simulink model "twolevel_parallel"  (R2016a)
settings: Solver=VariableStepAuto  StartTime=0.0  StopTime=stop_time  RelTol=1e-3
values from neighbouring files (symbols this model uses):
  DCLINK_Cap = 0.6*capacitorsabiti/sw_frequency    (= 0.0016)    [loadvariation.m]    (also in twolevel_parallel_analysis.m = 0.0001)
  Ef = Vln_rms*cos(Load_Angle)    [loadvariation.m]    (also in twolevel_parallel_analysis.m)
  intangle1 = 0    [loadvariation.m]    (also in twolevel_parallel_analysis.m)
  intangle2 = intangle1 + interleaving_angle    (= 360)    [loadvariation.m]    (also in twolevel_parallel_analysis.m = 180)
  Load_Angle = acos(Load_Power_Factor)    [loadvariation.m]    (also in twolevel_parallel_analysis.m)
  Ls = Xs/ref_frequency    [loadvariation.m]    (also in twolevel_parallel_analysis.m = n*Xs/ref_frequency)
  ma = 0.9    [loadvariation.m]    (also in twolevel_parallel_analysis.m)
  ref_frequency = 2*pi*50    (= 314.159265359)    [loadvariation.m]    (also in twolevel_parallel_analysis.m)
  Sampling_time = 1/(20*50000)    (= 1e-06)    [loadvariation.m]    (also in twolevel_parallel_analysis.m = 2.43902439024e-05)
  Vin = DC_Voltage_Source + Rin*(Load_Real_Power/DC_Voltage_Source)    (= 554.814814815)    [loadvariation.m]    (also in twolevel_parallel_analysis.m)
undefined symbols (not defined in the file or in its folder): Rload
libraries: powerlib x37, powerlib_meascontrol x23, simulink x12
settings Model: Creator=hakan  LastModifiedBy=hakan

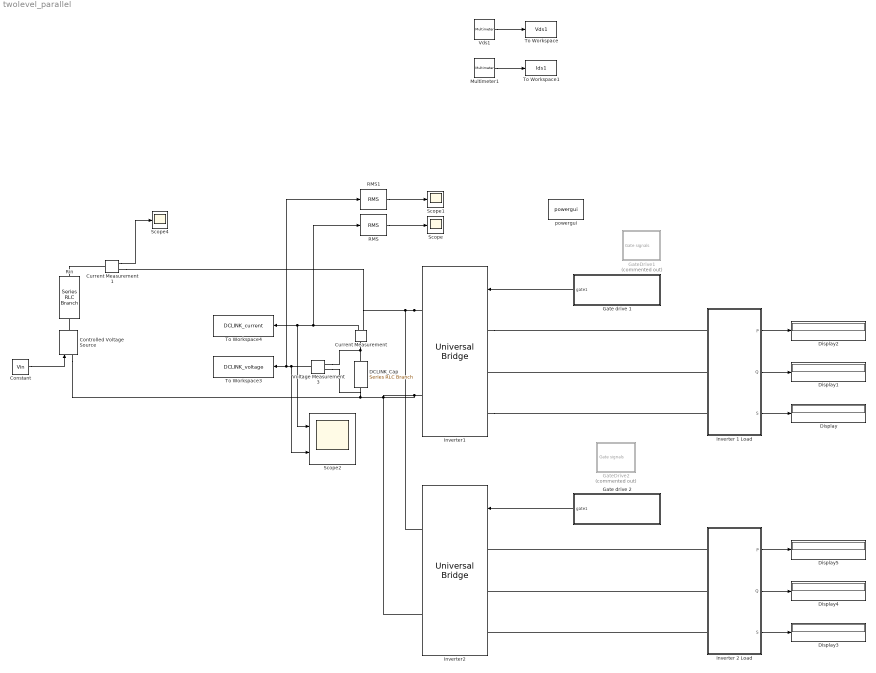
== system twolevel_parallel ==
  Constant : Constant  Value=Vin
  Controlled Voltage Source : powerlib/Electrical Sources/Controlled Voltage Source  Initialize=on  Source_Type=DC  Amplitude=0  Phase=0  Frequency=0  Measurements=None
  Current Measurement : powerlib/Measurements/Current Measurement  PhasorSimulation=off  OutputType=Complex  PSBequivalent=0
  Current Measurement1 : powerlib/Measurements/Current Measurement  PhasorSimulation=off  OutputType=Complex  PSBequivalent=0
  DCLINK_Cap : powerlib/Elements/Series RLC Branch  LConnTagsString=__new0  RConnTagsString=__new0  BranchType=C  Resistance=1  Inductance=1e-3  SetiL0=off  InitialCurrent=0  Capacitance=DCLINK_Cap  Setx0=on  InitialVoltage=540  Measurements=None
  Display{,1..5} (6 alike) : Display
  Gate drive 1 : Subsystem
  Gate drive 2 : Subsystem
  GateDrive1 : Subsystem  Commented=on
  GateDrive2 : Subsystem  Commented=on
  Inverter 1 Load : Subsystem
  Inverter 2 Load : Subsystem
  Inverter1 : powerlib/Power Electronics/Universal Bridge  Arms=3  SnubberResistance=1e5  SnubberCapacitance=inf  Device=IGBT / Diodes  Ron=0.65e-3  Lon=0  ForwardVoltages="[  0  0  ]"  ForwardVoltage=0  GTOparameters=[ 10e-6 , 20e-6 ]  IGBTparameters=[ 1e-6 , 2e-6 ]  Measurements=All voltages and currents  Measurements_2=None  converterType=Rectifier
  Inverter2 : powerlib/Power Electronics/Universal Bridge  Arms=3  SnubberResistance=1e5  SnubberCapacitance=inf  Device=IGBT / Diodes  Ron=0.65e-3  Lon=0  ForwardVoltages="[  0  0  ]"  ForwardVoltage=0  GTOparameters=[ 10e-6 , 20e-6 ]  IGBTparameters=[ 1e-6 , 2e-6 ]  Measurements=All voltages and currents  Measurements_2=None  converterType=Rectifier
  Multimeter1 : powerlib/Measurements/Multimeter  PhasorSimulation=off  OutputType=Complex  sel=27  L=32  Gain=1  yselected={'Isw1: Inverter1'};  PSBOutputType=1  PSBequivalent=0  AxesSetting=[0,0.1,-100,100]  Display=0  SavedBlockNames=-11
  RMS : powerlib_meascontrol/Measurements/RMS  TrueRMS=on  Freq=Load_Nominal_Freq  RMSInit=10  Ts=0
  RMS1 : powerlib_meascontrol/Measurements/RMS  TrueRMS=on  Freq=Load_Nominal_Freq  RMSInit=10  Ts=0
  Rin : powerlib/Elements/Series RLC Branch  LConnTagsString=__new0  RConnTagsString=__new0  BranchType=R  Resistance=1  Inductance=1e-3  SetiL0=off  InitialCurrent=0  Capacitance=1000e-6  Setx0=off  InitialVoltage=0  Measurements=None
  Scope : Scope
  Scope1 : Scope
  Scope2 : Scope  NumInputPorts=2
  Scope4 : Scope
  To Workspace : ToWorkspace  VariableName=Vds1  SaveFormat=Timeseries  SampleTime=-1
  To Workspace1 : ToWorkspace  VariableName=Ids1  SaveFormat=Timeseries  SampleTime=-1
  To Workspace3 : ToWorkspace  VariableName=DCLINK_voltage  SaveFormat=Timeseries  SampleTime=-1
  To Workspace4 : ToWorkspace  VariableName=DCLINK_current  SaveFormat=Timeseries  SampleTime=-1
  Vds1 : powerlib/Measurements/Multimeter  PhasorSimulation=off  OutputType=Complex  sel=11  L=32  Gain=1  yselected={'Usw1: Inverter1'};  PSBOutputType=1  PSBequivalent=0  AxesSetting=[0,0.1,-100,100]  Display=0  SavedBlockNames=-11
  Voltage Measurement3 : powerlib/Measurements/Voltage Measurement  PhasorSimulation=off  OutputType=Complex  PSBequivalent=0
  powergui : powerlib/powergui  Priority=1  SimulationMode=Discrete  SolverType=Tustin  SampleTime=Sampling_time  frequency=60  SPID=off  DisableSnubberDevices=off  DisableRonSwitches=off  DisableVfSwitches=off  SwTol=0  DisplayEquations=off  Interpol=off  ExternalGateDelay=off  methode=off  Ts=10  FunctionMessages=off  echomessages=off  HookPort=off  EnableUseOfTLC=off  x0status=blocks  frequencyindice=0  Pbase=100e6  ErrMax=1e-4  Iterations=50  UnitsV=kV  UnitsW=MW  buscounter=0  RestoreLinks=warning  ResistiveCurrentMeasurement=off  Frange=[0:2:500]  Ylog=off  Xlog=on  ShowGrid=off  save=off  variable=ZData  structure=Phase_currents  ZoomFFT=off  StartTime=0.1  cycles=5  DisplayStyle=1  fundamental=50  FreqAxis=off  MaxFrequency=2000  frequencyindicesteady=1  RmsSteady=1  display=off
  wires:
  Constant/1 -> Controlled Voltage Source/1
  Current Measurement/1 -> Scope2/1, To Workspace4/1, RMS/1
  Voltage Measurement3/1 -> Scope2/2, RMS1/1, To Workspace3/1
  Gate drive 2/1(gate1) -> Inverter2/1
  RMS/1 -> Scope/1
  RMS1/1 -> Scope1/1
  Current Measurement1/1 -> Scope4/1
  Gate drive 1/1(gate1) -> Inverter1/1
  Inverter 1 Load/1(P) -> Display2/1
  Inverter 1 Load/2(Q) -> Display1/1
  Inverter 1 Load/3(S) -> Display/1
  Inverter 2 Load/1(P) -> Display5/1
  Inverter 2 Load/2(Q) -> Display4/1
  Inverter 2 Load/3(S) -> Display3/1
  Multimeter1/1 -> To Workspace1/1
  Vds1/1 -> To Workspace/1
  connections:
  Controlled Voltage Source/RConn1 -- Rin/RConn1
  Inverter1/RConn1 -- Inverter2/RConn1 -- Current Measurement1/RConn1 -- Current Measurement/RConn1
  Inverter1/RConn2 -- Inverter2/RConn2 -- Controlled Voltage Source/LConn1 -- DCLINK_Cap/RConn1 -- Voltage Measurement3/LConn2
  Current Measurement/LConn1 -- DCLINK_Cap/LConn1 -- Voltage Measurement3/LConn1
  Inverter1/LConn1 -- Inverter 1 Load/LConn1
  Inverter 1 Load/LConn2 -- Inverter1/LConn2
  Inverter1/LConn3 -- Inverter 1 Load/LConn3
  Inverter 2 Load/LConn1 -- Inverter2/LConn1
  Inverter 2 Load/LConn3 -- Inverter2/LConn3
  Inverter 2 Load/LConn2 -- Inverter2/LConn2
  Rin/LConn1 -- Current Measurement1/LConn1

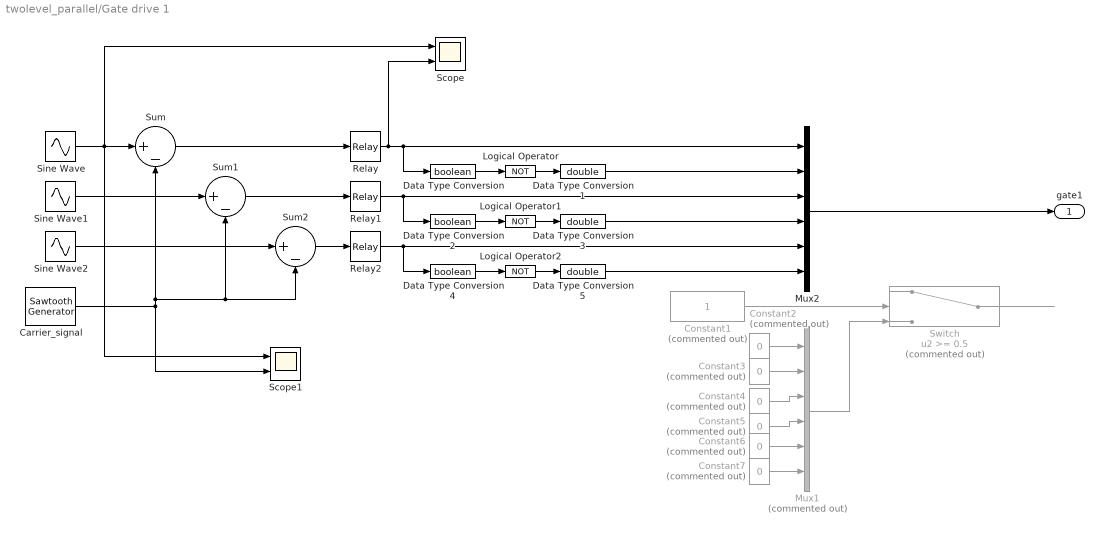
== system twolevel_parallel/Gate drive 1 ==
  Carrier_signal : powerlib_meascontrol/Pulse & Signal Generators/Sawtooth Generator  Freq=sw_frequency  Phase=intangle1  Ts=0
  Constant1 : Constant  Commented=on
  Constant{2..7} (6 alike) : Constant  Commented=on  Value=0
  Data Type Conversion : DataTypeConversion  OutDataTypeStr=boolean
  Data Type Conversion1 : DataTypeConversion  OutDataTypeStr=double
  Data Type Conversion2 : DataTypeConversion  OutDataTypeStr=boolean
  Data Type Conversion3 : DataTypeConversion  OutDataTypeStr=double
  Data Type Conversion4 : DataTypeConversion  OutDataTypeStr=boolean
  Data Type Conversion5 : DataTypeConversion  OutDataTypeStr=double
  Logical Operator : Logic  Operator=NOT  AllPortsSameDT=off  OutDataTypeStr=boolean
  Logical Operator1 : Logic  Operator=NOT  AllPortsSameDT=off  OutDataTypeStr=boolean
  Logical Operator2 : Logic  Operator=NOT  AllPortsSameDT=off  OutDataTypeStr=boolean
  Mux1 : Mux  Commented=on  Inputs=6
  Mux2 : Mux  Inputs=6
  Relay : Relay
  Relay1 : Relay
  Relay2 : Relay
  Scope : Scope  NumInputPorts=2
  Scope1 : Scope  NumInputPorts=2
  Sine Wave : Sin  Amplitude=ma  Frequency=ref_frequency  Phase=Load_Angle  SampleTime=0
  Sine Wave1 : Sin  Amplitude=ma  Frequency=ref_frequency  Phase=-2*pi/3+Load_Angle  SampleTime=0
  Sine Wave2 : Sin  Amplitude=ma  Frequency=ref_frequency  Phase=2*pi/3+Load_Angle  SampleTime=0
  Sum : Sum  Inputs=|+-
  Sum1 : Sum  Inputs=|+-
  Sum2 : Sum  Inputs=|+-
  Switch : Switch  Commented=on  Threshold=0.5
  gate1 : Outport
  wires:
  Sine Wave/1 -> Scope1/1, Scope/1, Sum/1
  Carrier_signal/1 -> Sum1/2, Sum2/2, Sum/2, Scope1/2
  Sine Wave1/1 -> Sum1/1
  Sine Wave2/1 -> Sum2/1
  Sum/1 -> Relay/1
  Sum1/1 -> Relay1/1
  Sum2/1 -> Relay2/1
  Data Type Conversion/1 -> Logical Operator/1
  Relay/1 -> Scope/2, Data Type Conversion/1, Mux2/1
  Logical Operator/1 -> Data Type Conversion1/1
  Data Type Conversion1/1 -> Mux2/2
  Data Type Conversion2/1 -> Logical Operator1/1
  Relay1/1 -> Data Type Conversion2/1, Mux2/3
  Logical Operator1/1 -> Data Type Conversion3/1
  Data Type Conversion3/1 -> Mux2/4
  Data Type Conversion4/1 -> Logical Operator2/1
  Relay2/1 -> Data Type Conversion4/1, Mux2/5
  Logical Operator2/1 -> Data Type Conversion5/1
  Data Type Conversion5/1 -> Mux2/6
  Constant1/1 -> Switch/2
  Constant2/1 -> Mux1/1
  Constant3/1 -> Mux1/2
  Constant4/1 -> Mux1/3
  Constant5/1 -> Mux1/4
  Constant7/1 -> Mux1/6
  Constant6/1 -> Mux1/5
  Mux1/1 -> Switch/3
  Switch/1 -> ?
  Mux2/1 -> gate1/1

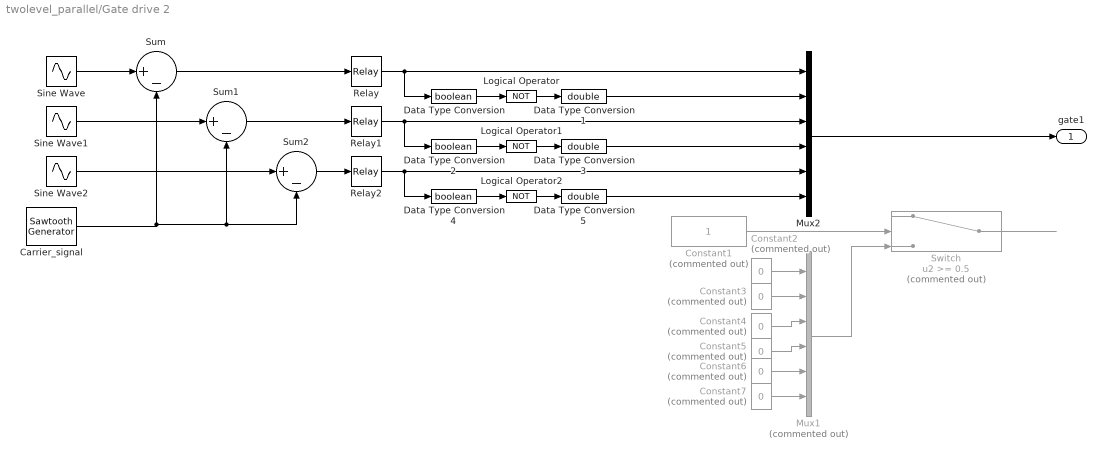
== system twolevel_parallel/Gate drive 2 ==
  Carrier_signal : powerlib_meascontrol/Pulse & Signal Generators/Sawtooth Generator  Freq=sw_frequency  Phase=intangle2  Ts=0
  Constant1 : Constant  Commented=on
  Constant{2..7} (6 alike) : Constant  Commented=on  Value=0
  Data Type Conversion : DataTypeConversion  OutDataTypeStr=boolean
  Data Type Conversion1 : DataTypeConversion  OutDataTypeStr=double
  Data Type Conversion2 : DataTypeConversion  OutDataTypeStr=boolean
  Data Type Conversion3 : DataTypeConversion  OutDataTypeStr=double
  Data Type Conversion4 : DataTypeConversion  OutDataTypeStr=boolean
  Data Type Conversion5 : DataTypeConversion  OutDataTypeStr=double
  Logical Operator : Logic  Operator=NOT  AllPortsSameDT=off  OutDataTypeStr=boolean
  Logical Operator1 : Logic  Operator=NOT  AllPortsSameDT=off  OutDataTypeStr=boolean
  Logical Operator2 : Logic  Operator=NOT  AllPortsSameDT=off  OutDataTypeStr=boolean
  Mux1 : Mux  Commented=on  Inputs=6
  Mux2 : Mux  Inputs=6
  Relay : Relay
  Relay1 : Relay
  Relay2 : Relay
  Sine Wave : Sin  Amplitude=ma  Frequency=ref_frequency  Phase=Load_Angle  SampleTime=0
  Sine Wave1 : Sin  Amplitude=ma  Frequency=ref_frequency  Phase=-2*pi/3+Load_Angle  SampleTime=0
  Sine Wave2 : Sin  Amplitude=ma  Frequency=ref_frequency  Phase=2*pi/3+Load_Angle  SampleTime=0
  Sum : Sum  Inputs=|+-
  Sum1 : Sum  Inputs=|+-
  Sum2 : Sum  Inputs=|+-
  Switch : Switch  Commented=on  Threshold=0.5
  gate1 : Outport
  wires:
  Mux2/1 -> gate1/1
  Switch/1 -> ?
  Mux1/1 -> Switch/3
  Constant6/1 -> Mux1/5
  Constant7/1 -> Mux1/6
  Constant5/1 -> Mux1/4
  Constant4/1 -> Mux1/3
  Constant3/1 -> Mux1/2
  Constant2/1 -> Mux1/1
  Constant1/1 -> Switch/2
  Data Type Conversion5/1 -> Mux2/6
  Logical Operator2/1 -> Data Type Conversion5/1
  Relay2/1 -> Mux2/5, Data Type Conversion4/1
  Data Type Conversion4/1 -> Logical Operator2/1
  Data Type Conversion3/1 -> Mux2/4
  Logical Operator1/1 -> Data Type Conversion3/1
  Relay1/1 -> Mux2/3, Data Type Conversion2/1
  Data Type Conversion2/1 -> Logical Operator1/1
  Data Type Conversion1/1 -> Mux2/2
  Logical Operator/1 -> Data Type Conversion1/1
  Relay/1 -> Mux2/1, Data Type Conversion/1
  Data Type Conversion/1 -> Logical Operator/1
  Sum2/1 -> Relay2/1
  Sum1/1 -> Relay1/1
  Sum/1 -> Relay/1
  Sine Wave2/1 -> Sum2/1
  Sine Wave1/1 -> Sum1/1
  Carrier_signal/1 -> Sum/2, Sum2/2, Sum1/2
  Sine Wave/1 -> Sum/1

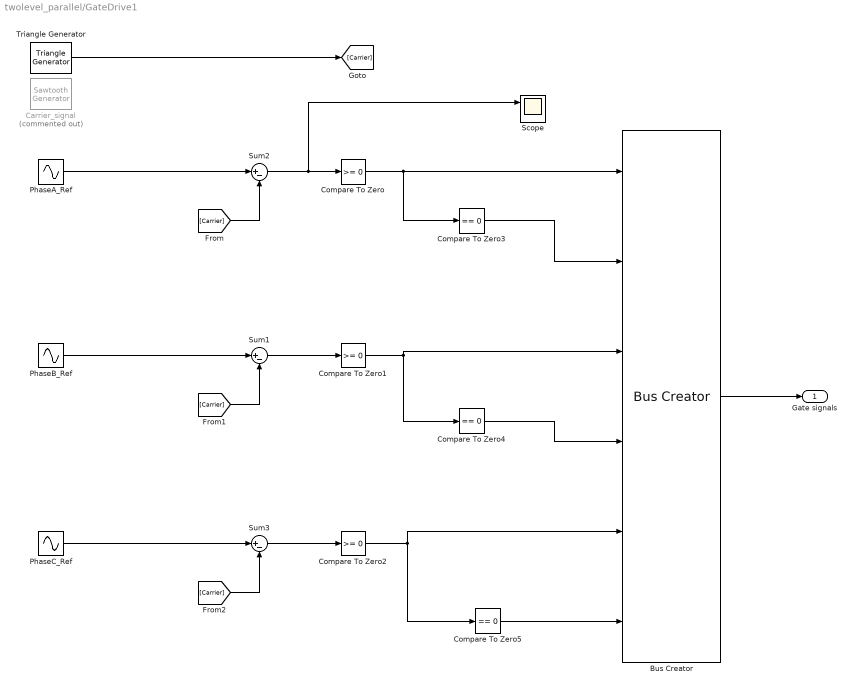
== system twolevel_parallel/GateDrive1 ==
  Bus Creator : BusCreator  Inputs=6
  Carrier_signal : powerlib_meascontrol/Pulse & Signal Generators/Sawtooth Generator  Commented=on  Freq=sw_frequency  Phase=intangle1  Ts=0
  Compare To Zero : simulink/Logic and Bit Operations/Compare To Zero  relop=>=  OutDataTypeStr=boolean  ZeroCross=off
  Compare To Zero1 : simulink/Logic and Bit Operations/Compare To Zero  relop=>=  OutDataTypeStr=boolean  ZeroCross=off
  Compare To Zero2 : simulink/Logic and Bit Operations/Compare To Zero  relop=>=  OutDataTypeStr=boolean  ZeroCross=off
  Compare To Zero3 : simulink/Logic and Bit Operations/Compare To Zero  relop===  OutDataTypeStr=boolean  ZeroCross=off
  Compare To Zero4 : simulink/Logic and Bit Operations/Compare To Zero  relop===  OutDataTypeStr=boolean  ZeroCross=off
  Compare To Zero5 : simulink/Logic and Bit Operations/Compare To Zero  relop===  OutDataTypeStr=boolean  ZeroCross=off
  PhaseA_Ref : Sin  Amplitude=ma  Frequency=ref_frequency  Phase=Load_Angle  SampleTime=0
  PhaseB_Ref : Sin  Amplitude=ma  Frequency=ref_frequency  Phase=-2*pi/3 + Load_Angle  SampleTime=0
  PhaseC_Ref : Sin  Amplitude=ma  Frequency=ref_frequency  Phase=2*pi/3+Load_Angle  SampleTime=0
  Scope : Scope  NumInputPorts=2
  Sum1 : Sum  Inputs=|+-
  Sum2 : Sum  Inputs=|+-
  Sum3 : Sum  Inputs=|+-
  Triangle Generator : powerlib_meascontrol/Pulse & Signal Generators/Triangle Generator  Freq=sw_frequency  Phase=intangle1  Ts=0
  Gate signals : Outport
  wires:
  Triangle Generator/1 -> [Carrier]
  Compare To Zero5/1 -> Bus Creator/6
  Compare To Zero4/1 -> Bus Creator/4
  Compare To Zero3/1 -> Bus Creator/2
  Sum3/1 -> Compare To Zero2/1
  Sum1/1 -> Compare To Zero1/1
  [Carrier] -> Sum3/2
  PhaseC_Ref/1 -> Sum3/1
  Compare To Zero2/1 -> Bus Creator/5, Compare To Zero5/1
  [Carrier] -> Sum1/2
  PhaseB_Ref/1 -> Sum1/1
  Compare To Zero1/1 -> Bus Creator/3, Compare To Zero4/1
  [Carrier] -> Sum2/2
  Sum2/1 -> Scope/1, Compare To Zero/1
  Compare To Zero/1 -> Bus Creator/1, Compare To Zero3/1
  PhaseA_Ref/1 -> Sum2/1
  Bus Creator/1 -> Gate signals/1

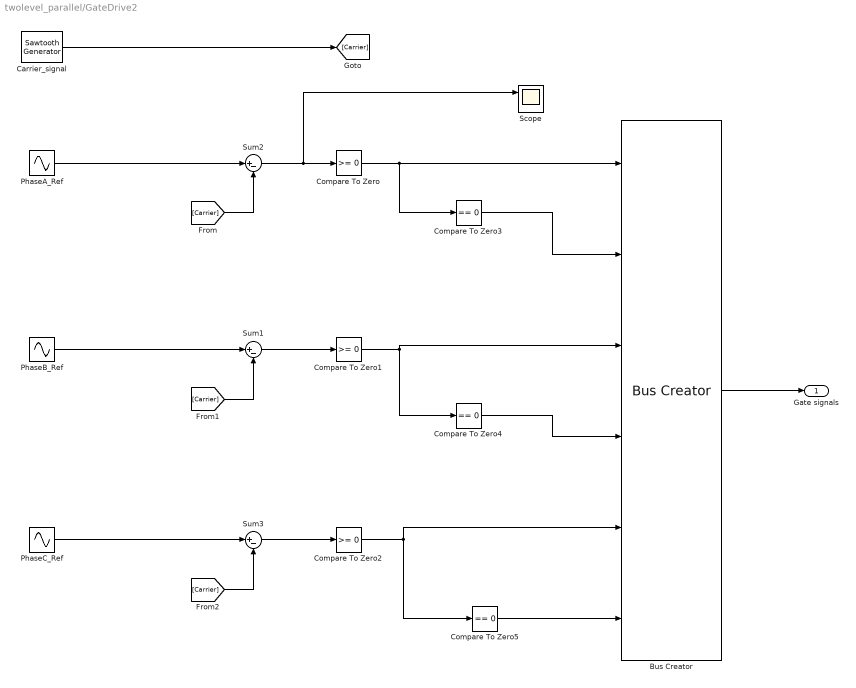
== system twolevel_parallel/GateDrive2 ==
  Bus Creator : BusCreator  Inputs=6
  Carrier_signal : powerlib_meascontrol/Pulse & Signal Generators/Sawtooth Generator  Freq=sw_frequency  Phase=intangle1  Ts=0
  Compare To Zero : simulink/Logic and Bit Operations/Compare To Zero  relop=>=  OutDataTypeStr=boolean  ZeroCross=off
  Compare To Zero1 : simulink/Logic and Bit Operations/Compare To Zero  relop=>=  OutDataTypeStr=boolean  ZeroCross=off
  Compare To Zero2 : simulink/Logic and Bit Operations/Compare To Zero  relop=>=  OutDataTypeStr=boolean  ZeroCross=off
  Compare To Zero3 : simulink/Logic and Bit Operations/Compare To Zero  relop===  OutDataTypeStr=boolean  ZeroCross=off
  Compare To Zero4 : simulink/Logic and Bit Operations/Compare To Zero  relop===  OutDataTypeStr=boolean  ZeroCross=off
  Compare To Zero5 : simulink/Logic and Bit Operations/Compare To Zero  relop===  OutDataTypeStr=boolean  ZeroCross=off
  PhaseA_Ref : Sin  Amplitude=ma  Frequency=ref_frequency  SampleTime=0
  PhaseB_Ref : Sin  Amplitude=ma  Frequency=ref_frequency  Phase=-2*pi/3  SampleTime=0
  PhaseC_Ref : Sin  Amplitude=ma  Frequency=ref_frequency  Phase=2*pi/3  SampleTime=0
  Scope : Scope  NumInputPorts=2
  Sum1 : Sum  Inputs=|+-
  Sum2 : Sum  Inputs=|+-
  Sum3 : Sum  Inputs=|+-
  Gate signals : Outport
  wires:
  Bus Creator/1 -> Gate signals/1
  PhaseA_Ref/1 -> Sum2/1
  Compare To Zero/1 -> Compare To Zero3/1, Bus Creator/1
  Sum2/1 -> Compare To Zero/1, Scope/1
  [Carrier] -> Sum2/2
  Compare To Zero1/1 -> Compare To Zero4/1, Bus Creator/3
  PhaseB_Ref/1 -> Sum1/1
  [Carrier] -> Sum1/2
  Compare To Zero2/1 -> Compare To Zero5/1, Bus Creator/5
  PhaseC_Ref/1 -> Sum3/1
  [Carrier] -> Sum3/2
  Sum1/1 -> Compare To Zero1/1
  Sum3/1 -> Compare To Zero2/1
  Compare To Zero3/1 -> Bus Creator/2
  Compare To Zero4/1 -> Bus Creator/4
  Compare To Zero5/1 -> Bus Creator/6
  Carrier_signal/1 -> [Carrier]

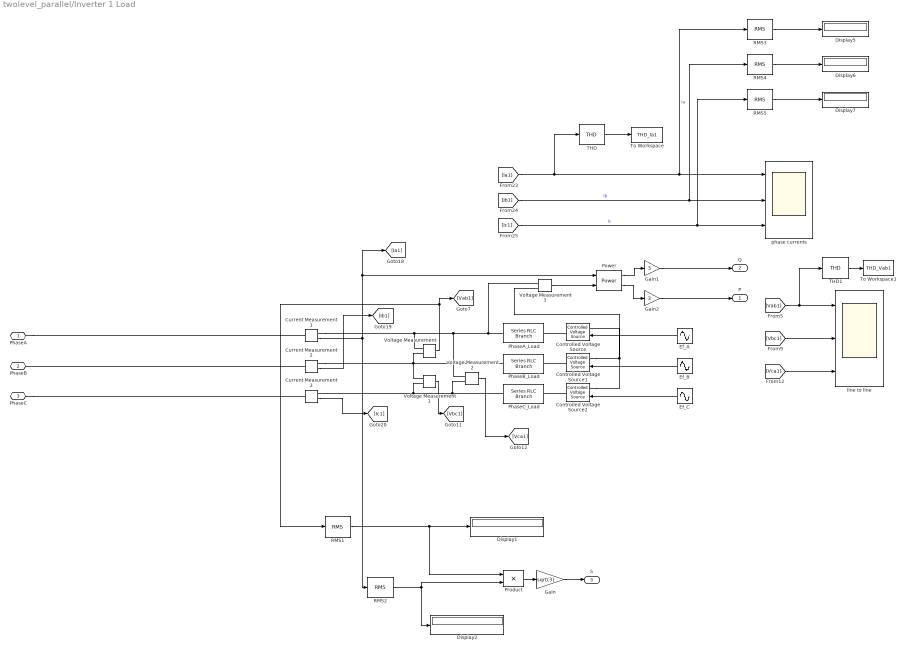
== system twolevel_parallel/Inverter 1 Load ==
  Controlled Voltage Source : powerlib/Electrical Sources/Controlled Voltage Source  Initialize=on  Source_Type=AC  Amplitude=0  Phase=0  Frequency=0  Measurements=None
  Controlled Voltage Source1 : powerlib/Electrical Sources/Controlled Voltage Source  Initialize=on  Source_Type=AC  Amplitude=0  Phase=0  Frequency=0  Measurements=None
  Controlled Voltage Source2 : powerlib/Electrical Sources/Controlled Voltage Source  Initialize=on  Source_Type=AC  Amplitude=0  Phase=0  Frequency=0  Measurements=None
  Current Measurement1 : powerlib/Measurements/Current Measurement  PhasorSimulation=off  OutputType=Complex  PSBequivalent=0
  Current Measurement2 : powerlib/Measurements/Current Measurement  PhasorSimulation=off  OutputType=Complex  PSBequivalent=0
  Current Measurement3 : powerlib/Measurements/Current Measurement  PhasorSimulation=off  OutputType=Complex  PSBequivalent=0
  Display{1..2,5..7} (5 alike) : Display
  Ef_A : Sin  Amplitude=Ef*sqrt(2)  Frequency=ref_frequency  SampleTime=0
  Ef_B : Sin  Amplitude=Ef*sqrt(2)  Frequency=ref_frequency  Phase=-2*pi/3  SampleTime=0
  Ef_C : Sin  Amplitude=Ef*sqrt(2)  Frequency=ref_frequency  Phase=2*pi/3  SampleTime=0
  Gain : Gain  Gain=sqrt(3)
  Gain1 : Gain  Gain=3
  Gain2 : Gain  Gain=3
  PhaseA_Load : powerlib/Elements/Series RLC Branch  LConnTagsString=__new0  RConnTagsString=__new0  BranchType=L  Resistance=Rload  Inductance=Ls  SetiL0=off  InitialCurrent=0  Capacitance=1e-6  Setx0=off  InitialVoltage=0  Measurements=None
  PhaseB_Load : powerlib/Elements/Series RLC Branch  LConnTagsString=__new0  RConnTagsString=__new0  BranchType=L  Resistance=Rload  Inductance=Ls  SetiL0=off  InitialCurrent=0  Capacitance=1e-6  Setx0=off  InitialVoltage=0  Measurements=None
  PhaseC_Load : powerlib/Elements/Series RLC Branch  LConnTagsString=__new0  RConnTagsString=__new0  BranchType=L  Resistance=Rload  Inductance=Ls  SetiL0=off  InitialCurrent=0  Capacitance=1e-6  Setx0=off  InitialVoltage=0  Measurements=None
  Power : powerlib_meascontrol/Measurements/Power  Freq=50  Vinit=[1, 0]  Iinit=[1, 0]  Ts=0
  Product : Product
  RMS1 : powerlib_meascontrol/Measurements/RMS  TrueRMS=off  Freq=Load_Nominal_Freq  RMSInit=120  Ts=0
  RMS{2..5} (4 alike) : powerlib_meascontrol/Measurements/RMS  TrueRMS=on  Freq=Load_Nominal_Freq  RMSInit=120  Ts=0
  THD : powerlib_meascontrol/Measurements/THD  Freq=50  Ts=0
  THD1 : powerlib_meascontrol/Measurements/THD  Freq=50  Ts=0
  To Workspace : ToWorkspace  VariableName=THD_Ia1  SaveFormat=Timeseries  SampleTime=-1
  To Workspace1 : ToWorkspace  VariableName=THD_Vab1  SaveFormat=Timeseries  SampleTime=-1
  Voltage Measurement{,1..3} (4 alike) : powerlib/Measurements/Voltage Measurement  PhasorSimulation=off  OutputType=Complex  PSBequivalent=0
  line to line : Scope  NumInputPorts=3
  phase currents : Scope  NumInputPorts=3
  PhaseA : PMIOPort  Port=1  Side=Left
  PhaseB : PMIOPort  Port=2  Side=Left
  PhaseC : PMIOPort  Port=3  Side=Left
  P : Outport
  Q : Outport  Port=2
  S : Outport  Port=3
  wires:
  Current Measurement2/1 -> [Ib1]
  Voltage Measurement/1 -> [Vab1], RMS1/1
  Voltage Measurement1/1 -> [Vbc1]
  Current Measurement3/1 -> [Ic1]
  [Ia1] -> THD/1, RMS3/1, phase currents/1  "Ia"
  [Ic1] -> RMS5/1, phase currents/3  "Ic"
  [Vbc1] -> line to line/2
  [Vab1] -> THD1/1, line to line/1
  [Vca1] -> line to line/3
  THD/1 -> To Workspace/1
  Voltage Measurement2/1 -> [Vca1]
  [Ib1] -> RMS4/1, phase currents/2  "Ib"
  THD1/1 -> To Workspace1/1
  Product/1 -> Gain/1
  RMS1/1 -> Product/1, Display1/1
  RMS2/1 -> Product/2, Display2/1
  Gain/1 -> S/1
  Power/2 -> Gain1/1
  Power/1 -> Gain2/1
  Voltage Measurement3/1 -> Power/1
  Gain1/1 -> Q/1
  Gain2/1 -> P/1
  RMS3/1 -> Display5/1
  RMS4/1 -> Display6/1
  RMS5/1 -> Display7/1
  Current Measurement1/1 -> [Ia1], Power/2, RMS2/1
  Ef_A/1 -> Controlled Voltage Source/1
  Ef_B/1 -> Controlled Voltage Source1/1
  Ef_C/1 -> Controlled Voltage Source2/1
  connections:
  Current Measurement2/RConn1 -- Voltage Measurement1/LConn1 -- Voltage Measurement/LConn2 -- PhaseB_Load/LConn1
  PhaseC/RConn1 -- Current Measurement3/LConn1
  PhaseC_Load/LConn1 -- Voltage Measurement2/LConn1 -- Voltage Measurement1/LConn2 -- Current Measurement3/RConn1
  Current Measurement2/LConn1 -- PhaseB/RConn1
  PhaseA/RConn1 -- Current Measurement1/LConn1
  Current Measurement1/RConn1 -- Voltage Measurement/LConn1 -- Voltage Measurement2/LConn2 -- Voltage Measurement3/LConn1 -- PhaseA_Load/LConn1
  Controlled Voltage Source1/LConn1 -- Controlled Voltage Source2/LConn1 -- Voltage Measurement3/LConn2 -- Controlled Voltage Source/LConn1
  Controlled Voltage Source1/RConn1 -- PhaseB_Load/RConn1
  Controlled Voltage Source/RConn1 -- PhaseA_Load/RConn1
  Controlled Voltage Source2/RConn1 -- PhaseC_Load/RConn1

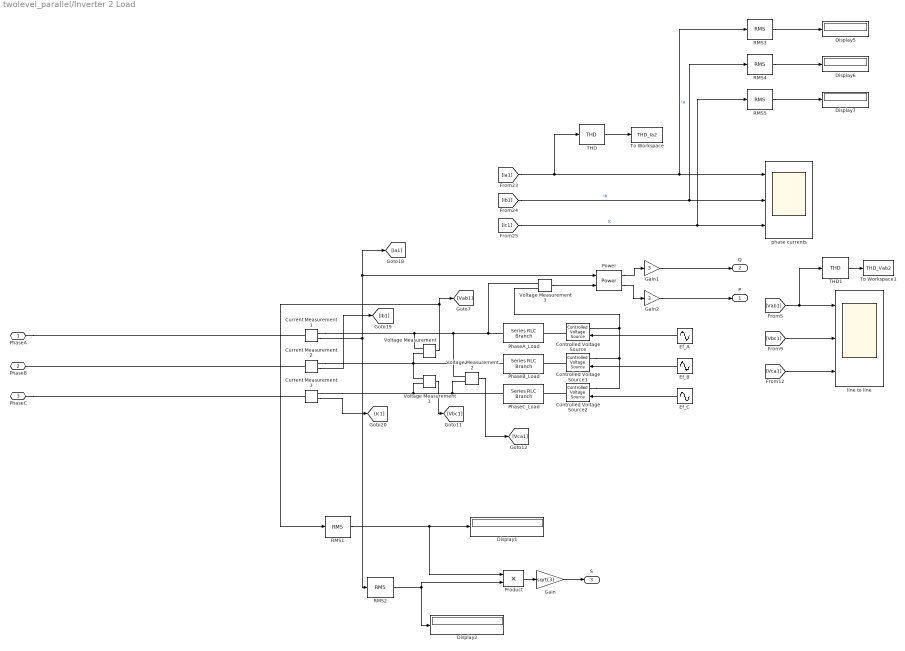
== system twolevel_parallel/Inverter 2 Load ==
  Controlled Voltage Source : powerlib/Electrical Sources/Controlled Voltage Source  Initialize=on  Source_Type=AC  Amplitude=0  Phase=0  Frequency=0  Measurements=None
  Controlled Voltage Source1 : powerlib/Electrical Sources/Controlled Voltage Source  Initialize=on  Source_Type=AC  Amplitude=0  Phase=0  Frequency=0  Measurements=None
  Controlled Voltage Source2 : powerlib/Electrical Sources/Controlled Voltage Source  Initialize=on  Source_Type=AC  Amplitude=0  Phase=0  Frequency=0  Measurements=None
  Current Measurement1 : powerlib/Measurements/Current Measurement  PhasorSimulation=off  OutputType=Complex  PSBequivalent=0
  Current Measurement2 : powerlib/Measurements/Current Measurement  PhasorSimulation=off  OutputType=Complex  PSBequivalent=0
  Current Measurement3 : powerlib/Measurements/Current Measurement  PhasorSimulation=off  OutputType=Complex  PSBequivalent=0
  Display{1..2,5..7} (5 alike) : Display
  Ef_A : Sin  Amplitude=Ef*sqrt(2)  Frequency=ref_frequency  SampleTime=0
  Ef_B : Sin  Amplitude=Ef*sqrt(2)  Frequency=ref_frequency  Phase=-2*pi/3  SampleTime=0
  Ef_C : Sin  Amplitude=Ef*sqrt(2)  Frequency=ref_frequency  Phase=2*pi/3  SampleTime=0
  Gain : Gain  Gain=sqrt(3)
  Gain1 : Gain  Gain=3
  Gain2 : Gain  Gain=3
  PhaseA_Load : powerlib/Elements/Series RLC Branch  LConnTagsString=__new0  RConnTagsString=__new0  BranchType=L  Resistance=Rload  Inductance=Ls  SetiL0=off  InitialCurrent=0  Capacitance=1e-6  Setx0=off  InitialVoltage=0  Measurements=None
  PhaseB_Load : powerlib/Elements/Series RLC Branch  LConnTagsString=__new0  RConnTagsString=__new0  BranchType=L  Resistance=Rload  Inductance=Ls  SetiL0=off  InitialCurrent=0  Capacitance=1e-6  Setx0=off  InitialVoltage=0  Measurements=None
  PhaseC_Load : powerlib/Elements/Series RLC Branch  LConnTagsString=__new0  RConnTagsString=__new0  BranchType=L  Resistance=Rload  Inductance=Ls  SetiL0=off  InitialCurrent=0  Capacitance=1e-6  Setx0=off  InitialVoltage=0  Measurements=None
  Power : powerlib_meascontrol/Measurements/Power  Freq=50  Vinit=[1, 0]  Iinit=[1, 0]  Ts=0
  Product : Product
  RMS1 : powerlib_meascontrol/Measurements/RMS  TrueRMS=off  Freq=Load_Nominal_Freq  RMSInit=120  Ts=0
  RMS{2..5} (4 alike) : powerlib_meascontrol/Measurements/RMS  TrueRMS=on  Freq=Load_Nominal_Freq  RMSInit=120  Ts=0
  THD : powerlib_meascontrol/Measurements/THD  Freq=50  Ts=0
  THD1 : powerlib_meascontrol/Measurements/THD  Freq=50  Ts=0
  To Workspace : ToWorkspace  VariableName=THD_Ia2  SaveFormat=Timeseries  SampleTime=-1
  To Workspace1 : ToWorkspace  VariableName=THD_Vab2  SaveFormat=Timeseries  SampleTime=-1
  Voltage Measurement{,1..3} (4 alike) : powerlib/Measurements/Voltage Measurement  PhasorSimulation=off  OutputType=Complex  PSBequivalent=0
  line to line : Scope  NumInputPorts=3
  phase currents : Scope  NumInputPorts=3
  PhaseA : PMIOPort  Port=1  Side=Left
  PhaseB : PMIOPort  Port=2  Side=Left
  PhaseC : PMIOPort  Port=3  Side=Left
  P : Outport
  Q : Outport  Port=2
  S : Outport  Port=3
  wires:
  Ef_C/1 -> Controlled Voltage Source2/1
  Ef_B/1 -> Controlled Voltage Source1/1
  Ef_A/1 -> Controlled Voltage Source/1
  Current Measurement1/1 -> RMS2/1, Power/2, [Ia1]
  RMS5/1 -> Display7/1
  RMS4/1 -> Display6/1
  RMS3/1 -> Display5/1
  Gain2/1 -> P/1
  Gain1/1 -> Q/1
  Voltage Measurement3/1 -> Power/1
  Power/1 -> Gain2/1
  Power/2 -> Gain1/1
  Gain/1 -> S/1
  RMS2/1 -> Display2/1, Product/2
  RMS1/1 -> Display1/1, Product/1
  Product/1 -> Gain/1
  THD1/1 -> To Workspace1/1
  [Ib1] -> phase currents/2, RMS4/1  "Ib"
  Voltage Measurement2/1 -> [Vca1]
  THD/1 -> To Workspace/1
  [Vca1] -> line to line/3
  [Vab1] -> line to line/1, THD1/1
  [Vbc1] -> line to line/2
  [Ic1] -> phase currents/3, RMS5/1  "Ic"
  [Ia1] -> phase currents/1, RMS3/1, THD/1  "Ia"
  Current Measurement3/1 -> [Ic1]
  Voltage Measurement1/1 -> [Vbc1]
  Voltage Measurement/1 -> RMS1/1, [Vab1]
  Current Measurement2/1 -> [Ib1]
  connections:
  Controlled Voltage Source2/RConn1 -- PhaseC_Load/RConn1
  Controlled Voltage Source/RConn1 -- PhaseA_Load/RConn1
  Controlled Voltage Source1/RConn1 -- PhaseB_Load/RConn1
  Controlled Voltage Source/LConn1 -- Voltage Measurement3/LConn2 -- Controlled Voltage Source1/LConn1 -- Controlled Voltage Source2/LConn1
  PhaseA_Load/LConn1 -- Voltage Measurement3/LConn1 -- Voltage Measurement2/LConn2 -- Voltage Measurement/LConn1 -- Current Measurement1/RConn1
  PhaseA/RConn1 -- Current Measurement1/LConn1
  Current Measurement2/LConn1 -- PhaseB/RConn1
  Current Measurement3/RConn1 -- Voltage Measurement1/LConn2 -- Voltage Measurement2/LConn1 -- PhaseC_Load/LConn1
  PhaseC/RConn1 -- Current Measurement3/LConn1
  PhaseB_Load/LConn1 -- Voltage Measurement/LConn2 -- Voltage Measurement1/LConn1 -- Current Measurement2/RConn1
